simulink model "STATCOM_ssc_Ccode"  (R2024b)
settings: Solver=FixedStepDiscrete  StartTime=0.0  StopTime=2  FixedStep=Ts  RelTol=1e-3  EnableMultiTasking=on
PostLoadFcn:
  | Ts=25e-6; Rsnu=500; Csnu=0.1e-6;
InitFcn:
  | Ts=25e-6; Rsnu=500; Csnu=0.1e-6;
undefined symbols (not defined in the file): DiscIntNeverNeededParam
libraries: ee_lib x19, simetran x14, fl_lib x12, nesl_utility x12, spsSecondOrderFilterLib x3, spsabctodq0Lib x2, simulink x1, spsMeanVariableFrequencyLib x1
(part 2 of 3)

== system STATCOM_ssc_Ccode/STATCOM Controller/Firing Pulses Generator ==
  Alpha : Inport  PortDimensions=1
  Sigma : Inport  Port=2  PortDimensions=1
  wt : Inport  Port=3  PortDimensions=1
  D_Alpha : Inport  Port=4  PortDimensions=1
  " Deg->Rad" : Gain  Gain=pi/180  SaturateOnIntegerOverflow=on  OutDataTypeStr=Inherit: Same as input  ParamDataTypeStr=Inherit: Same as input
  Bridge 1D : Subsystem
  "Bridge 1Y " : Subsystem
  Bridge 2D : Subsystem
  Bridge 2Y : Subsystem
  Constant : Constant  Value=[0 -30 -15 -45]*pi/180 + 7.5*pi/180
  Deg->Rad : Gain  Gain=pi/180  SaturateOnIntegerOverflow=on  OutDataTypeStr=Inherit: Same as input  ParamDataTypeStr=Inherit: Same as input
  "Deg->Rad " : Gain  Gain=pi/180  SaturateOnIntegerOverflow=on  OutDataTypeStr=Inherit: Same as input  ParamDataTypeStr=Inherit: Same as input
  Demux : Demux
      settings: DisplayOption=none
  Mux : Mux  Inputs=[12 12 12 12]
  Sum : Sum  InputSameDT=on  SaturateOnIntegerOverflow=on  OutDataTypeStr=Inherit: Same as first input
  Pulses : Outport  VectorParamsAs1DForOutWhenUnconnected=off
  wires:
  wt/1 -> Sum/1
  Bridge 2D/1(Pulses) -> Mux/4
  Bridge 2Y/1(Pulses) -> Mux/3
  Bridge 1D/1(Pulses) -> Mux/2
  D_Alpha/1 -> " Deg->Rad"/1
  " Deg->Rad"/1 -> "Bridge 1Y "/4(D_Alpha), Bridge 1D/4(D_Alpha), Bridge 2Y/4(D_Alpha), Bridge 2D/4(D_Alpha)
  "Deg->Rad "/1 -> Bridge 2D/3(Sigma), Bridge 2Y/3(Sigma), Bridge 1D/3(Sigma), "Bridge 1Y "/3(Sigma)
  Deg->Rad/1 -> Bridge 2D/2(Alpha), Bridge 2Y/2(Alpha), Bridge 1D/2(Alpha), "Bridge 1Y "/2(Alpha)
  Demux/4 -> Bridge 2D/1(wt)
  Demux/3 -> Bridge 2Y/1(wt)
  Demux/2 -> Bridge 1D/1(wt)
  Sigma/1 -> "Deg->Rad "/1
  Demux/1 -> "Bridge 1Y "/1(wt)
  Mux/1 -> Pulses/1
  "Bridge 1Y "/1(Pulses) -> Mux/1
  Sum/1 -> Demux/1
  Constant/1 -> Sum/2
  Alpha/1 -> Deg->Rad/1

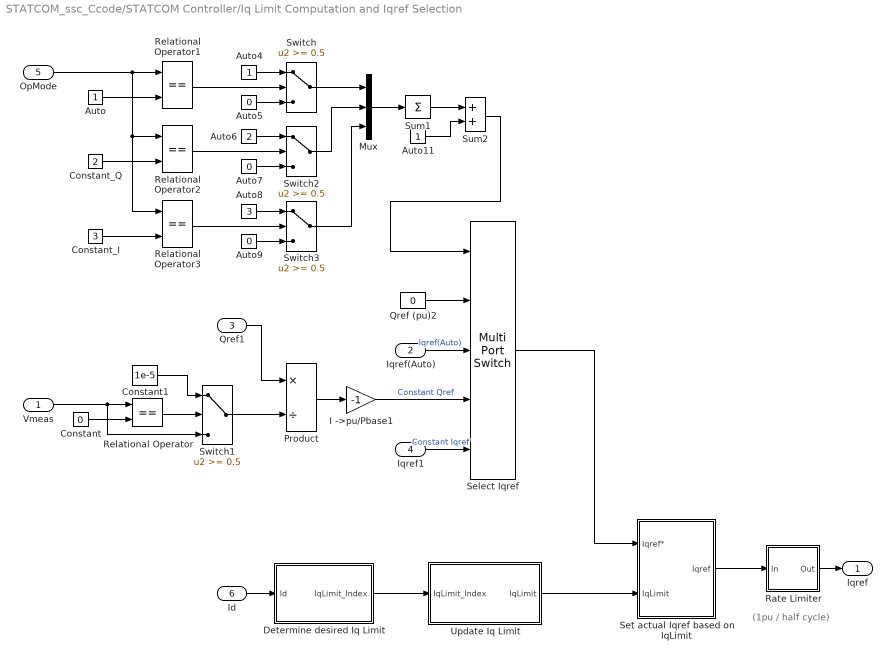
== system STATCOM_ssc_Ccode/STATCOM Controller/Iq Limit Computation and Iqref Selection ==
  note: (1pu / half cycle)
  Vmeas : Inport
  Iqref(Auto) : Inport  Port=2
  Qref1 : Inport  Port=3
  Iqref1 : Inport  Port=4
  OpMode : Inport  Port=5
  Id : Inport  Port=6
  Auto : Constant
  Auto11 : Constant
  Auto4 : Constant
  Auto5 : Constant  Value=0
  Auto6 : Constant  Value=2
  Auto7 : Constant  Value=0
  Auto8 : Constant  Value=3
  Auto9 : Constant  Value=0
  Constant : Constant  Value=0
  Constant1 : Constant  Value=1e-5
  Constant_I : Constant  Value=3
  Constant_Q : Constant  Value=2
  Determine desired Iq Limit : Subsystem
  I ->pu/Pbase1 : Gain  Gain=-1  SaturateOnIntegerOverflow=on  OutDataTypeStr=Inherit: Same as input  ParamDataTypeStr=Inherit: Same as input
  Mux : Mux  Inputs=3
  Product : Product  Inputs=*/  InputSameDT=on  SaturateOnIntegerOverflow=on  OutDataTypeStr=Inherit: Same as first input
  Qref (pu)2 : Constant  Value=0
  "Rate Limiter " : Subsystem  DialogController=POWERSYS.PowerSysDialog  mask(Discrete Rate Limiter){R=120, F=-120, Vinit=-0.33, Ts=Ts}
      mask prompts: R "Rising slew rate:"; F "Falling slew rate:"; Vinit "Initial input:"; Ts "Sample time:"
      mask help: DISCRETE BLOCK : Limit rising and falling rates of signal
      mask init:
      | UpperLimit=R*Ts;
      | LowerLimit=F*Ts;
      | power_initmask();
      mask Help: This block is part of a subset of blocks in the Extras library that does not have documentation associated with it, other than the block mask description.
      mask Display: disp('Discrete\nRate\nLimiter')
  Relational Operator{,1..3} (4 alike) : RelationalOperator  Operator===
  Select Iqref : MultiPortSwitch  Inputs=4
  Set actual Iqref based on IqLimit : Subsystem
  Sum1 : Sum  Inputs=1  InputSameDT=on  SaturateOnIntegerOverflow=on  OutDataTypeStr=Inherit: Same as first input
  Sum2 : Sum  InputSameDT=on  SaturateOnIntegerOverflow=on  OutDataTypeStr=Inherit: Same as first input
  Switch{,1..3} (4 alike) : Switch  Threshold=0.5
  Update Iq Limit : Subsystem
  Iqref : Outport  VectorParamsAs1DForOutWhenUnconnected=off
  wires:
  Id/1 -> Determine desired Iq Limit/1(Id)
  "Rate Limiter "/1(Out) -> Iqref/1
  Update Iq Limit/1(IqLimit) -> Set actual Iqref based on IqLimit/2(IqLimit)
  Determine desired Iq Limit/1(IqLimit_Index) -> Update Iq Limit/1(IqLimit_Index)
  Select Iqref/1 -> Set actual Iqref based on IqLimit/1(Iqref*)
  Qref (pu)2/1 -> Select Iqref/2
  I ->pu/Pbase1/1 -> Select Iqref/4  "Constant Qref"
  Iqref(Auto)/1 -> Select Iqref/3  "Iqref(Auto)"
  Iqref1/1 -> Select Iqref/5  "Constant Iqref"
  Product/1 -> I ->pu/Pbase1/1
  Constant/1 -> Relational Operator/2
  Switch1/1 -> Product/2
  Constant1/1 -> Switch1/1
  Relational Operator/1 -> Switch1/2
  Qref1/1 -> Product/1
  Vmeas/1 -> Switch1/3, Relational Operator/1
  Sum2/1 -> Select Iqref/1
  Auto/1 -> Relational Operator1/2
  Constant_Q/1 -> Relational Operator2/2
  Constant_I/1 -> Relational Operator3/2
  OpMode/1 -> Relational Operator1/1, Relational Operator2/1, Relational Operator3/1
  Relational Operator1/1 -> Switch/2
  Auto4/1 -> Switch/1
  Auto5/1 -> Switch/3
  Relational Operator2/1 -> Switch2/2
  Auto6/1 -> Switch2/1
  Auto7/1 -> Switch2/3
  Relational Operator3/1 -> Switch3/2
  Auto8/1 -> Switch3/1
  Auto9/1 -> Switch3/3
  Switch/1 -> Mux/1
  Mux/1 -> Sum1/1
  Switch3/1 -> Mux/3
  Sum1/1 -> Sum2/1
  Auto11/1 -> Sum2/2
  Switch2/1 -> Mux/2
  Set actual Iqref based on IqLimit/1(Iqref) -> "Rate Limiter "/1(In)

== system STATCOM_ssc_Ccode/STATCOM Controller/Measurement System ==
  Vabc : Inport  PortDimensions=3
  Iabc : Inport  Port=2  PortDimensions=3
  Freq : Inport  Port=3  PortDimensions=1
  wt : Inport  Port=4  PortDimensions=1
  Mean value : Subsystem  mask(Discrete Variable-Frequency Mean Value){Finit=60, Vinit=0, Ts=Ts}
      mask prompts: Finit "Initial Frequency (Hz):"; Vinit "Initial input (DC component):"; Ts "Sample time:"
      mask help:
      | This discrete block computes the mean value of the input signal (port In) over a running window of one cycle of a specified frequency (port Freq).
      |
      | For the first cycle of simulation (specified by the parameter "Initial frequency"), the output is held to the value of the  "Initial input" parameter.
  Mux : Mux  Inputs=2
  PQ Computaion : Subsystem
  Reactive current measurement (Iq) : Subsystem  mask(abc to dq0 Transformation){}
      mask help:
      | This block performs the  abc to dq0 transformation on a set of three-phase signals.
      |
      | It computes the three components ( Vd=direct axis , Vq=quadrature axis and V0=zero sequence) in a two axis rotating reference frame according to the following transformation:
      |
      | Vd = 2/3*[Va*sin(wt)  + Vb*sin(wt-2pi/3)  +  Vc*sin(wt+2pi/3)]
      | Vq = 2/3*[Va*cos(wt) + Vb*cos(wt-2pi/3) + Vc*cos(wt+2pi/3)]
      | V0 = 1/3*[Va +  Vb  +  Vc ]
      | where w=  rotation speed (rad/s) of the rotating frame.
      |
      | Input 1 contains  the vectorized  signals of the three  [Va Vb  Vc] sinusoidal phase quantities.
      | Input 2 must contain a  [sin(wt)  cos(wt)] two dimension signal , where w is the rotation speed (rad/s)  of the reference frame.
      | Output is a vectozized signal containing the [Vd Vq Vo] components.
      |
      | Press Help for more information.
      mask Help:
      | This transformation is commonly used in three-phase electric machine models where it is known as Park transformation. It allows to eliminate time varying inductances by referring the stator and rotor quantities to a fixed or rotating reference frame .
      | In case of a synchrounous machine, the stator quantities are referred to the rotor. Id and Iq represent the two DC currents flowing  in the two equivalent rotor windings ( d winding on the same axis as the field winding, and q winding in quadrature) producing the same flux as the stator Ia, Ib and Ic currents.
      | 
      | You can also use this block in a control system to measure the positive-sequence component V1 of a set of three-phase voltages or currents.
      | Vd and Vq represent the rectangular coordinates of  V1.
      | Use the Math Function block (hypot) and the Trigonometric function block (atan2) to obtain the modulus and angle of V1.
      | Mag(V1) = sqrt(Vd^2 + Vq^2);
      | Phase(V1)=atan2(Vq/Vd).
      | This measurement system does not introduce any delay, but, in contrast with the Fourier analysis (See Sequence Analyzer block), it is sensitive to harmonics and unbalances.
      | 
      | See also the dq0_to_abc block performing the reverse transformation.
  Second-Order Filter : spsSecondOrderFilterLib/Second-Order Filter  FilterType=Lowpass  Fo=1200  Zeta=0.707  Ts=Ts  Initialize=off  Vac_Init="[0,  0,  60]"  Vdc_Init=0  PlotResponse=off  FreqRange=[0, 500, 1]
  Second-Order Filter1 : spsSecondOrderFilterLib/Second-Order Filter  FilterType=Lowpass  Fo=1200  Zeta=0.707  Ts=Ts  Initialize=off  Vac_Init="[0,  0,  60]"  Vdc_Init=0  PlotResponse=off  FreqRange=[0, 500, 1]
  Selector : Selector  InputPortWidth=2  IndexOptions=Index vector (dialog)  Indices=2  OutputSizes=1
  Selector1 : Selector  InputPortWidth=2  IndexOptions=Index vector (dialog)  Indices=1  OutputSizes=1
  Trigonometric Function : Trigonometry
  Trigonometric Function1 : Trigonometry  Operator=cos
  Voltage measurement (Positive sequence) : Subsystem  mask(Discrete 3-phase PLL-Driven Positive-Sequence Fundamental Value){Finit=60, Par_Init=[1 0], Ts=Ts}
      mask prompts: Finit "Initial fundamental frequency (Hz):"; Par_Init "Initial input (positive component): [ Mag  Phase-relative-to-PLL(degrees) ]"; Ts "Sample time:"
      mask help:
      | For a supplied fundamental frequency (port Freq), this discrete block computes  the positive-sequence component (Magnitude and Phase)  of a set of three balanced or unbalanced signals (port abc) which may contain harmonics.
      |  Input port "Sin_Cos" (a two-dimension signal) provides the reference frame required for the computation..
      |  First and second outputs return respectively the magnitude and phase (in degrees relative to the PLL phase)) of the fundamental.
      | For the first cycle of simulation, the outputs are held constant to the values specified by the parameter "Initial input".
      mask init:
      | Real_Init=Par_Init(1)*cos(pi/180*Par_Init(2));
      | Imag_Init=Par_Init(1)*sin(pi/180*Par_Init(2));
  Vmeas : Outport  VectorParamsAs1DForOutWhenUnconnected=off
  PQ : Outport  Port=2  VectorParamsAs1DForOutWhenUnconnected=off
  Iq : Outport  Port=3  VectorParamsAs1DForOutWhenUnconnected=off
  Iq_avg : Outport  Port=4  VectorParamsAs1DForOutWhenUnconnected=off
  Id : Outport  Port=5  VectorParamsAs1DForOutWhenUnconnected=off
  wires:
  Second-Order Filter1/1 -> Iq/1
  Voltage measurement (Positive sequence)/2(VdVq) -> PQ Computaion/1(Vd_Vq)
  Voltage measurement (Positive sequence)/1(Mag) -> Vmeas/1  "Vmes"
  Vabc/1 -> Voltage measurement (Positive sequence)/1(abc)
  Trigonometric Function/1 -> Mux/1
  Trigonometric Function1/1 -> Mux/2
  wt/1 -> Trigonometric Function/1, Trigonometric Function1/1, Voltage measurement (Positive sequence)/3(wt)
  Iabc/1 -> Reactive current measurement (Iq)/2(abc)
  Mux/1 -> Reactive current measurement (Iq)/1(sin_cos)
  PQ Computaion/1(PQ(pu)) -> PQ/1
  Reactive current measurement (Iq)/1(IdIq) -> PQ Computaion/2(Id_Iq), Selector/1, Selector1/1
  Freq/1 -> Voltage measurement (Positive sequence)/2(Freq), PQ Computaion/3(Freq), Mean value/1(Freq)
  Selector/1 -> Mean value/2(In), Second-Order Filter1/1
  Mean value/1(Mean) -> Iq_avg/1
  Selector1/1 -> Second-Order Filter/1
  Second-Order Filter/1 -> Id/1

== system STATCOM_ssc_Ccode/STATCOM Controller/PLL ==
  Vabc (pu) : Inport  PortDimensions=3
  Constant4 : Constant  Value=2*pi
  Correction for delay : Gain  Gain=Nstep*Ts*2*pi  SaturateOnIntegerOverflow=on  OutDataTypeStr=Inherit: Same as input  ParamDataTypeStr=Inherit: Same as input
  Discrete PI Controller : Subsystem  DialogController=POWERSYS.PowerSysDialog  mask(Discrete PI Controller){Kp=Kp, Ki=Ki, Par_Limits=2*pi*Finit*[1.25 0.75], Init=2*pi*Finit, Ts=Ts}
      mask prompts: Kp "Proportional gain (Kp):"; Ki "Integral gain (Ki):"; Par_Limits "Output limits: [ Upper   Lower ]"; Init "Output initial value:"; Ts "Sample time:"
      mask help: This block implements a discrete PI controller.
      mask init:
      | UpperLimit=Par_Limits(1);
      | LowerLimit=Par_Limits(2);
      | power_initmask();
      mask Help: This block is part of a subset of blocks in the Extras library that does not have documentation associated with it, other than the block mask description.
      mask Display: disp('PI');
  Discrete Rate Limiter : Subsystem  DialogController=POWERSYS.PowerSysDialog  mask(Discrete Rate Limiter){R=10, F=-10, Vinit=Finit, Ts=Ts}
      mask prompts: R "Rising slew rate:"; F "Falling slew rate:"; Vinit "Initial input:"; Ts "Sample time:"
      mask help: DISCRETE BLOCK : Limit rising and falling rates of signal
      mask init:
      | UpperLimit=R*Ts;
      | LowerLimit=F*Ts;
      | power_initmask();
      mask Help: This block is part of a subset of blocks in the Extras library that does not have documentation associated with it, other than the block mask description.
      mask Display: disp('Discrete\nRate\nLimiter')
  Discrete-Time Integrator : DiscreteIntegrator  InitialCondition=Phase_Init*pi/180  SampleTime=Ts  ICPrevOutput=DiscIntNeverNeededParam  ICPrevScaledInput=DiscIntNeverNeededParam
  Gain10 : Gain  Gain=1/2/pi  SaturateOnIntegerOverflow=on  OutDataTypeStr=Inherit: Same as input  ParamDataTypeStr=Inherit: Same as input
  Math Function : Math  Operator=mod  SignedPower=on
  Mean (Variable Frequency) : spsMeanVariableFrequencyLib/Mean (Variable Frequency)  Finit=Finit  Fmin=45  Vinit=0  Ts=Ts
  Second-Order Filter : spsSecondOrderFilterLib/Second-Order Filter  FilterType=Lowpass  Fo=25  Zeta=0.707  Ts=Ts  Initialize=on  Vac_Init=[0 -25 60]  Vdc_Init=Finit  PlotResponse=off  FreqRange=[0, 500, 1]
  Selector : Selector  InputPortWidth=3  IndexOptions=Index vector (dialog)  Indices=2  OutputSizes=1
  Sum : Sum  InputSameDT=on  SaturateOnIntegerOverflow=on  OutDataTypeStr=Inherit: Same as first input
  Unit Delay : UnitDelay  InitialCondition=Finit  SampleTime=Ts  HasFrameUpgradeWarning=on
  abc to dq0 : spsabctodq0Lib/abc to dq0  Alignment=90 degrees behind phase A axis
  Freq : Outport  VectorParamsAs1DForOutWhenUnconnected=off
  wt : Outport  Port=2  VectorParamsAs1DForOutWhenUnconnected=off
  wires:
  Correction for delay/1 -> Sum/1
  Mean (Variable Frequency)/1 -> Discrete PI Controller/1(Error)
  Vabc (pu)/1 -> abc to dq0/1
  abc to dq0/1 -> Selector/1
  Constant4/1 -> Math Function/2
  Discrete-Time Integrator/1 -> Math Function/1
  Math Function/1 -> Sum/2, abc to dq0/2
  Discrete PI Controller/1(Out) -> Discrete-Time Integrator/1, Gain10/1  "W"
  Gain10/1 -> Discrete Rate Limiter/1(In)
  Discrete Rate Limiter/1(Out) -> Second-Order Filter/1
  Unit Delay/1 -> Freq/1, Mean (Variable Frequency)/1, Correction for delay/1
  Second-Order Filter/1 -> Unit Delay/1
  Selector/1 -> Mean (Variable Frequency)/2  "Vq"
  Sum/1 -> wt/1

== system STATCOM_ssc_Ccode/STATCOM Controller/Voltage Regulator ==
  Vref : Inport
  Vmeas : Inport  Port=2
  Discrete-Time Integrator : DiscreteIntegrator  InitialCondition=Init  SampleTime=Ts  LimitOutput=on  UpperSaturationLimit=UpperLimit  LowerSaturationLimit=LowerLimit  ICPrevOutput=DiscIntNeverNeededParam  ICPrevScaledInput=DiscIntNeverNeededParam
  Kp4 : Gain  Gain=Kp  SaturateOnIntegerOverflow=on  OutDataTypeStr=Inherit: Same as input  ParamDataTypeStr=Inherit: Same as input
  Kp5 : Gain  Gain=Ki  SaturateOnIntegerOverflow=on  OutDataTypeStr=Inherit: Same as input  ParamDataTypeStr=Inherit: Same as input
  Kp6 : Gain  Gain=Droop  SaturateOnIntegerOverflow=on  OutDataTypeStr=Inherit: Same as input  ParamDataTypeStr=Inherit: Same as input
  Saturation2 : Saturate  UpperLimit=UpperLimit  LowerLimit=LowerLimit
  Sum1 : Sum  Inputs=|-+  InputSameDT=on  SaturateOnIntegerOverflow=on  OutDataTypeStr=Inherit: Same as first input
  Sum6 : Sum  InputSameDT=on  SaturateOnIntegerOverflow=on  OutDataTypeStr=Inherit: Same as first input
  Sum7 : Sum  Inputs=|+-  InputSameDT=on  SaturateOnIntegerOverflow=on  OutDataTypeStr=Inherit: Same as first input
  Unit Delay : UnitDelay  SampleTime=Ts  HasFrameUpgradeWarning=on
  Iqref : Outport  InitialOutput=0  VectorParamsAs1DForOutWhenUnconnected=off
  wires:
  Discrete-Time Integrator/1 -> Sum6/2
  Kp4/1 -> Sum6/1
  Sum6/1 -> Saturation2/1
  Kp5/1 -> Discrete-Time Integrator/1
  Sum7/1 -> Kp5/1, Kp4/1
  Saturation2/1 -> Iqref/1, Kp6/1  "Iq_Ref"
  Kp6/1 -> Unit Delay/1
  Unit Delay/1 -> Sum7/2
  Vmeas/1 -> Sum1/1
  Vref/1 -> Sum1/2
  Sum1/1 -> Sum7/1  "Err"

== system STATCOM_ssc_Ccode/STATCOM Controller/DC Balance Regulator/ Mean value ==
  note: Discrete Mean Value
  note: Pierre Giroux, Gilbert Sybille
      | Power System Simulation Laboratory
      | IREQ, Hydro-Quebc
  In : Inport
  Constant : Constant  Value=Vinit
  Constant1 : Constant  Value=Correction
  Integ4 : DiscreteIntegrator  IntegratorMethod=Integration: Trapezoidal  SampleTime=Ts  ICPrevOutput=DiscIntNeverNeededParam  ICPrevScaledInput=DiscIntNeverNeededParam
  K2 : Constant  Value=Freq
  Product : Product  InputSameDT=on  SaturateOnIntegerOverflow=on  OutDataTypeStr=Inherit: Same as first input
  Product1 : Product  Inputs=**  InputSameDT=on  SaturateOnIntegerOverflow=on  OutDataTypeStr=Inherit: Same as first input
  Step : Step  Time=1/Freq  SampleTime=Ts
  Sum5 : Sum  InputSameDT=on  SaturateOnIntegerOverflow=on  OutDataTypeStr=Inherit: Same as first input
  Sum7 : Sum  Inputs=-+  InputSameDT=on  SaturateOnIntegerOverflow=on  OutDataTypeStr=Inherit: Same as first input
  Switch : Switch  Threshold=0.5
  Transport Delay : TransportDelay  DelayTime=Delay
  Mean : Outport  VectorParamsAs1DForOutWhenUnconnected=off
  wires:
  Switch/1 -> Mean/1
  Constant/1 -> Switch/3
  Step/1 -> Switch/2
  Sum5/1 -> Switch/1
  Product1/1 -> Sum5/2  "Correction"
  Constant1/1 -> Product1/2
  In/1 -> Product1/1, Integ4/1  "In"
  K2/1 -> Product/2
  Integ4/1 -> Sum7/2, Transport Delay/1
  Sum7/1 -> Product/1
  Transport Delay/1 -> Sum7/1
  Product/1 -> Sum5/1  "Mean value"

== system STATCOM_ssc_Ccode/STATCOM Controller/DC Balance Regulator/PI Regulator ==
  note: Discrete PID Controller
  note: Pierre Giroux, Gilbert Sybille
      | Power System Simulation Laboratory
      | IREQ, Hydro-Quebc
  Error : Inport
  Reset : Inport  Port=2
  Discrete-Time Integrator : DiscreteIntegrator  ExternalReset=rising  InitialCondition=Init  SampleTime=Ts  LimitOutput=on  UpperSaturationLimit=UpperLimit  LowerSaturationLimit=LowerLimit  ICPrevOutput=DiscIntNeverNeededParam  ICPrevScaledInput=DiscIntNeverNeededParam
  Kp4 : Gain  Gain=Kp  SaturateOnIntegerOverflow=on  OutDataTypeStr=Inherit: Same as input  ParamDataTypeStr=Inherit: Same as input
  Kp5 : Gain  Gain=Ki  SaturateOnIntegerOverflow=on  OutDataTypeStr=Inherit: Same as input  ParamDataTypeStr=Inherit: Same as input
  Saturation2 : Saturate  UpperLimit=UpperLimit  LowerLimit=LowerLimit
  Sum6 : Sum  InputSameDT=on  SaturateOnIntegerOverflow=on  OutDataTypeStr=Inherit: Same as first input
  Out : Outport  InitialOutput=0  VectorParamsAs1DForOutWhenUnconnected=off
  wires:
  Reset/1 -> Discrete-Time Integrator/2
  Error/1 -> Kp4/1, Kp5/1
  Sum6/1 -> Saturation2/1
  Kp5/1 -> Discrete-Time Integrator/1
  Kp4/1 -> Sum6/1
  Discrete-Time Integrator/1 -> Sum6/2
  Saturation2/1 -> Out/1

== system STATCOM_ssc_Ccode/STATCOM Controller/Firing Pulses Generator/Bridge 1D ==
  wt : Inport  PortDimensions=1
  Alpha : Inport  Port=2  PortDimensions=1
  Sigma : Inport  Port=3  PortDimensions=1
  D_Alpha : Inport  Port=4  PortDimensions=1
  Constant : Constant  Value=-2*pi/3
  Constant1 : Constant  Value=2*pi/3
  Mux1 : Mux  Inputs=[4 4 4]
  Phase A : Subsystem
  Phase B : Subsystem
  Phase C : Subsystem
  Sum : Sum  InputSameDT=on  SaturateOnIntegerOverflow=on  OutDataTypeStr=Inherit: Same as first input
  Sum1 : Sum  InputSameDT=on  SaturateOnIntegerOverflow=on  OutDataTypeStr=Inherit: Same as first input
  Sum2 : Sum  InputSameDT=on  SaturateOnIntegerOverflow=on  OutDataTypeStr=Inherit: Same as first input
  Pulses : Outport  VectorParamsAs1DForOutWhenUnconnected=off
  wires:
  Phase C/1(Pulses) -> Mux1/3
  Phase B/1(Pulses) -> Mux1/2
  D_Alpha/1 -> Phase C/3(D_Alpha), Phase B/3(D_Alpha), Phase A/3(D_Alpha)
  Sum1/1 -> Phase C/1(wt)
  Sum/1 -> Phase B/1(wt)
  Constant/1 -> Sum/2
  Phase A/1(Pulses) -> Mux1/1
  Mux1/1 -> Pulses/1
  Sum2/1 -> Sum1/1, Sum/1, Phase A/1(wt)
  wt/1 -> Sum2/1
  Alpha/1 -> Sum2/2
  Sigma/1 -> Phase B/2(sigma), Phase C/2(sigma), Phase A/2(sigma)
  Constant1/1 -> Sum1/2

== system STATCOM_ssc_Ccode/STATCOM Controller/Firing Pulses Generator/Bridge 1Y  ==
  wt : Inport  PortDimensions=1
  Alpha : Inport  Port=2  PortDimensions=1
  Sigma : Inport  Port=3  PortDimensions=1
  D_Alpha : Inport  Port=4  PortDimensions=1
  Constant : Constant  Value=-2*pi/3
  Constant1 : Constant  Value=2*pi/3
  Mux1 : Mux  Inputs=[4 4 4]
  Phase A : Subsystem
  Phase B : Subsystem
  Phase C : Subsystem
  Sum : Sum  InputSameDT=on  SaturateOnIntegerOverflow=on  OutDataTypeStr=Inherit: Same as first input
  Sum1 : Sum  InputSameDT=on  SaturateOnIntegerOverflow=on  OutDataTypeStr=Inherit: Same as first input
  Sum2 : Sum  InputSameDT=on  SaturateOnIntegerOverflow=on  OutDataTypeStr=Inherit: Same as first input
  Pulses : Outport  VectorParamsAs1DForOutWhenUnconnected=off
  wires:
  Constant1/1 -> Sum1/2
  Sigma/1 -> Phase A/2(sigma), Phase C/2(sigma), Phase B/2(sigma)
  Alpha/1 -> Sum2/2
  wt/1 -> Sum2/1
  Sum2/1 -> Phase A/1(wt), Sum/1, Sum1/1
  Mux1/1 -> Pulses/1
  Phase A/1(Pulses) -> Mux1/1
  Constant/1 -> Sum/2
  Sum/1 -> Phase B/1(wt)
  Sum1/1 -> Phase C/1(wt)
  D_Alpha/1 -> Phase A/3(D_Alpha), Phase B/3(D_Alpha), Phase C/3(D_Alpha)
  Phase B/1(Pulses) -> Mux1/2
  Phase C/1(Pulses) -> Mux1/3

== system STATCOM_ssc_Ccode/STATCOM Controller/Firing Pulses Generator/Bridge 2D ==
  wt : Inport  PortDimensions=1
  Alpha : Inport  Port=2  PortDimensions=1
  Sigma : Inport  Port=3  PortDimensions=1
  D_Alpha : Inport  Port=4  PortDimensions=1
  Constant : Constant  Value=-2*pi/3
  Constant1 : Constant  Value=2*pi/3
  Mux1 : Mux  Inputs=[4 4 4]
  Phase A : Subsystem
  Phase B : Subsystem
  Phase C : Subsystem
  Sum : Sum  InputSameDT=on  SaturateOnIntegerOverflow=on  OutDataTypeStr=Inherit: Same as first input
  Sum1 : Sum  InputSameDT=on  SaturateOnIntegerOverflow=on  OutDataTypeStr=Inherit: Same as first input
  Sum2 : Sum  InputSameDT=on  SaturateOnIntegerOverflow=on  OutDataTypeStr=Inherit: Same as first input
  Pulses : Outport  VectorParamsAs1DForOutWhenUnconnected=off
  wires:
  Phase C/1(Pulses) -> Mux1/3
  Phase B/1(Pulses) -> Mux1/2
  D_Alpha/1 -> Phase C/3(D_Alpha), Phase B/3(D_Alpha), Phase A/3(D_Alpha)
  Sum1/1 -> Phase C/1(wt)
  Sum/1 -> Phase B/1(wt)
  Constant/1 -> Sum/2
  Phase A/1(Pulses) -> Mux1/1
  Mux1/1 -> Pulses/1
  Sum2/1 -> Sum1/1, Sum/1, Phase A/1(wt)
  wt/1 -> Sum2/1
  Alpha/1 -> Sum2/2
  Sigma/1 -> Phase B/2(sigma), Phase C/2(sigma), Phase A/2(sigma)
  Constant1/1 -> Sum1/2

== system STATCOM_ssc_Ccode/STATCOM Controller/Firing Pulses Generator/Bridge 2Y ==
  wt : Inport  PortDimensions=1
  Alpha : Inport  Port=2  PortDimensions=1
  Sigma : Inport  Port=3  PortDimensions=1
  D_Alpha : Inport  Port=4  PortDimensions=1
  Constant : Constant  Value=-2*pi/3
  Constant1 : Constant  Value=2*pi/3
  Mux1 : Mux  Inputs=[4 4 4]
  Phase A : Subsystem
  Phase B : Subsystem
  Phase C : Subsystem
  Sum : Sum  InputSameDT=on  SaturateOnIntegerOverflow=on  OutDataTypeStr=Inherit: Same as first input
  Sum1 : Sum  InputSameDT=on  SaturateOnIntegerOverflow=on  OutDataTypeStr=Inherit: Same as first input
  Sum2 : Sum  InputSameDT=on  SaturateOnIntegerOverflow=on  OutDataTypeStr=Inherit: Same as first input
  Pulses : Outport  VectorParamsAs1DForOutWhenUnconnected=off
  wires:
  Constant1/1 -> Sum1/2
  Sigma/1 -> Phase A/2(sigma), Phase C/2(sigma), Phase B/2(sigma)
  Alpha/1 -> Sum2/2
  wt/1 -> Sum2/1
  Sum2/1 -> Phase A/1(wt), Sum/1, Sum1/1
  Mux1/1 -> Pulses/1
  Phase A/1(Pulses) -> Mux1/1
  Constant/1 -> Sum/2
  Sum/1 -> Phase B/1(wt)
  Sum1/1 -> Phase C/1(wt)
  D_Alpha/1 -> Phase A/3(D_Alpha), Phase B/3(D_Alpha), Phase C/3(D_Alpha)
  Phase B/1(Pulses) -> Mux1/2
  Phase C/1(Pulses) -> Mux1/3

== system STATCOM_ssc_Ccode/STATCOM Controller/Iq Limit Computation and Iqref Selection/Determine desired Iq Limit ==
  note: Determine desired Iq Limit (by step of 0.1 pu, from 1 to 0.3 pu)
      | based on actual value of Id
      | 5% above rated current is allowed
      | i.e.   sqrt ( Id^2 + Iq^2 ) < 1.05 pu
  Id : Inport  PortDimensions=1
  Abs : Abs
  Constant : Constant
  Limit at 0.3 : Relay  OnSwitchValue=0.97  OffSwitchValue=0.92
  Limit at 0.4 : Relay  OnSwitchValue=0.92  OffSwitchValue=0.86
  Limit at 0.5 : Relay  OnSwitchValue=0.86  OffSwitchValue=0.78
  Limit at 0.6 : Relay  OnSwitchValue=0.78  OffSwitchValue=0.68
  Limit at 0.7 : Relay  OnSwitchValue=0.68  OffSwitchValue=0.54
  Limit at 0.8 : Relay  OnSwitchValue=0.54  OffSwitchValue=0.32
  Limit at 0.9 : Relay  OnSwitchValue=0.32  OffSwitchValue=0.25
  Sum : Sum  Inputs=++++++++  InputSameDT=on  SaturateOnIntegerOverflow=on  OutDataTypeStr=Inherit: Same as first input
  IqLimit_Index : Outport  VectorParamsAs1DForOutWhenUnconnected=off
  wires:
  Sum/1 -> IqLimit_Index/1
  Limit at 0.9/1 -> Sum/2
  Limit at 0.8/1 -> Sum/3
  Limit at 0.7/1 -> Sum/4
  Limit at 0.6/1 -> Sum/5
  Constant/1 -> Sum/1
  Id/1 -> Abs/1
  Abs/1 -> Limit at 0.9/1, Limit at 0.8/1, Limit at 0.7/1, Limit at 0.6/1, Limit at 0.5/1, Limit at 0.4/1, Limit at 0.3/1
  Limit at 0.5/1 -> Sum/6
  Limit at 0.4/1 -> Sum/7
  Limit at 0.3/1 -> Sum/8

== system STATCOM_ssc_Ccode/STATCOM Controller/Iq Limit Computation and Iqref Selection/Rate Limiter  ==
  note: Delta(u)
  note: Beat Ronner
      | ABB Industrie AG
      | Turgi, Switzerland
  In : Inport
  Saturation : Saturate  UpperLimit=UpperLimit  LowerLimit=LowerLimit
  Sum : Sum  Inputs=|++  InputSameDT=on  SaturateOnIntegerOverflow=on  OutDataTypeStr=Inherit: Same as first input
  Sum1 : Sum  Inputs=|+-  InputSameDT=on  SaturateOnIntegerOverflow=on  OutDataTypeStr=Inherit: Same as first input
  Unit Delay : UnitDelay  InitialCondition=Vinit  SampleTime=Ts  HasFrameUpgradeWarning=on
  Out : Outport  VectorParamsAs1DForOutWhenUnconnected=off
  wires:
  In/1 -> Sum1/1  "u"
  Sum1/1 -> Saturation/1
  Saturation/1 -> Sum/1  "Delta(u)_limit"
  Sum/1 -> Out/1, Unit Delay/1  "y"
  Unit Delay/1 -> Sum1/2, Sum/2  "y-1"

== system STATCOM_ssc_Ccode/STATCOM Controller/Iq Limit Computation and Iqref Selection/Set actual Iqref based on IqLimit ==
  Iqref* : Inport  PortDimensions=1
  IqLimit : Inport  Port=2
  Gain2 : Gain  Gain=-1  SaturateOnIntegerOverflow=on  OutDataTypeStr=Inherit: Same as input  ParamDataTypeStr=Inherit: Same as input
  Logical Operator : Logic  Operator=OR
  Product : Product  InputSameDT=on  SaturateOnIntegerOverflow=on  OutDataTypeStr=Inherit: Same as first input
  Relational Operator1 : RelationalOperator  Operator=>
  Relational Operator2 : RelationalOperator  Operator=<
  Sign : Signum
  Switch1 : Switch  Threshold=0.5
  Iqref : Outport  VectorParamsAs1DForOutWhenUnconnected=off
  wires:
  Switch1/1 -> Iqref/1
  IqLimit/1 -> Product/1, Relational Operator1/2, Gain2/1
  Gain2/1 -> Relational Operator2/2
  Relational Operator1/1 -> Logical Operator/1
  Relational Operator2/1 -> Logical Operator/2
  Logical Operator/1 -> Switch1/2
  Iqref*/1 -> Relational Operator1/1, Relational Operator2/1, Switch1/3, Sign/1
  Sign/1 -> Product/2
  Product/1 -> Switch1/1

== system STATCOM_ssc_Ccode/STATCOM Controller/Iq Limit Computation and Iqref Selection/Update Iq Limit ==
  note: 2) Update of the new desired Iq limit is delayed by 3 cycles if the new desired limit is higher then the actual limit
  note: Rules for updating the Iq Limit in order to avoid control instability :
  note: 1) Instantaneous update of IqLimit if the new desired Iq limit is lower then the actual limit
  IqLimit_Index : Inport
  Constant1 : Constant  Value=0.8
  Constant10 : Constant  Value=-1e6
  Constant11 : Constant  Value=3
  Constant2 : Constant  Value=0.7
  Constant3 : Constant  Value=0.6
  Constant4 : Constant  Value=0.5
  Constant5 : Constant  Value=0.4
  Constant6 : Constant
  Constant7 : Constant  Value=0.9
  Constant8 : Constant  Value=0.3
  Constant9 : Constant  Value=60
  Discrete-Time Integrator : DiscreteIntegrator  ExternalReset=rising  SampleTime=Ts  LimitOutput=on  UpperSaturationLimit=6.1  LowerSaturationLimit=0  ICPrevOutput=DiscIntNeverNeededParam  ICPrevScaledInput=DiscIntNeverNeededParam
  Logical Operator1 : Logic  Operator=OR
  Relational Operator3 : RelationalOperator  Operator=>
  Relational Operator4 : RelationalOperator  Operator=>
  Relational Operator5 : RelationalOperator  Operator=<
  Select actual Iq Limit : MultiPortSwitch  Inputs=8
  Switch : Switch  Threshold=0.5
  Switch2 : Switch  Threshold=0.5
  Unit Delay : UnitDelay  SampleTime=Ts  HasFrameUpgradeWarning=on
  Unit Delay5 : UnitDelay  InitialCondition=1  SampleTime=Ts  HasFrameUpgradeWarning=on
  IqLimit : Outport  VectorParamsAs1DForOutWhenUnconnected=off
  wires:
  IqLimit_Index/1 -> Relational Operator5/2, Relational Operator3/2, Switch2/1
  Relational Operator5/1 -> Logical Operator1/2
  Relational Operator4/1 -> Logical Operator1/1, Unit Delay/1
  Discrete-Time Integrator/1 -> Relational Operator4/1
  Constant11/1 -> Relational Operator4/2
  Switch/1 -> Discrete-Time Integrator/1
  Unit Delay/1 -> Discrete-Time Integrator/2
  Constant9/1 -> Switch/1
  Constant10/1 -> Switch/3
  Relational Operator3/1 -> Switch/2
  Unit Delay5/1 -> Relational Operator5/1, Relational Operator3/1, Switch2/3, Select actual Iq Limit/1
  Switch2/1 -> Unit Delay5/1
  Logical Operator1/1 -> Switch2/2
  Select actual Iq Limit/1 -> IqLimit/1
  Constant3/1 -> Select actual Iq Limit/6
  Constant2/1 -> Select actual Iq Limit/5
  Constant1/1 -> Select actual Iq Limit/4
  Constant7/1 -> Select actual Iq Limit/3
  Constant6/1 -> Select actual Iq Limit/2
  Constant8/1 -> Select actual Iq Limit/9
  Constant5/1 -> Select actual Iq Limit/8
  Constant4/1 -> Select actual Iq Limit/7

== system STATCOM_ssc_Ccode/STATCOM Controller/Measurement System/Mean value ==
  note: Pierre Giroux, Gilbert Sybille
      | Power System Simulation Laboratory
      | IREQ, Hydro-Quebc
  note: Variable frequency - Discrete Mean Value
  Freq : Inport
  In : Inport  Port=2
  Constant : Constant  Value=Vinit
  Gain : Gain  Gain=Ts  SaturateOnIntegerOverflow=on  OutDataTypeStr=Inherit: Same as input  ParamDataTypeStr=Inherit: Same as input
  Integ4 : DiscreteIntegrator  IntegratorMethod=Integration: Trapezoidal  SampleTime=Ts  ICPrevOutput=DiscIntNeverNeededParam  ICPrevScaledInput=DiscIntNeverNeededParam
  K2 : Constant  Value=Ts/2
  Number of sample/cycle : Fcn  Expr=1/(u[1]+1e-6)/Ts
  Product : Product  InputSameDT=on  SaturateOnIntegerOverflow=on  OutDataTypeStr=Inherit: Same as first input
  Product1 : Product  Inputs=*/*  InputSameDT=on  SaturateOnIntegerOverflow=on  OutDataTypeStr=Inherit: Same as first input
  Rounding Function : Rounding  Operator=round
  Step : Step  Time=1/Finit  SampleTime=Ts
  Sum3 : Sum  Inputs=-+  InputSameDT=on  SaturateOnIntegerOverflow=on  OutDataTypeStr=Inherit: Same as first input
  Sum4 : Sum  Inputs=-+  InputSameDT=on  SaturateOnIntegerOverflow=on  OutDataTypeStr=Inherit: Same as first input
  Sum5 : Sum  InputSameDT=on  SaturateOnIntegerOverflow=on  OutDataTypeStr=Inherit: Same as first input
  Sum7 : Sum  Inputs=-+  InputSameDT=on  SaturateOnIntegerOverflow=on  OutDataTypeStr=Inherit: Same as first input
  Switch : Switch  Threshold=0.5
  Variable Transport Delay2 : VariableTransportDelay  MaximumDelay=20e-3
  Mean : Outport  VectorParamsAs1DForOutWhenUnconnected=off
  wires:
  Product1/1 -> Sum5/2  "Correction"
  In/1 -> Product1/3, Integ4/1  "In"
  Product/1 -> Sum5/1  "Mean value"
  Variable Transport Delay2/1 -> Sum7/1
  Sum7/1 -> Product/1
  Integ4/1 -> Variable Transport Delay2/1, Sum7/2
  Freq/1 -> Product/2, Number of sample/cycle/1  "Freq"
  K2/1 -> Sum3/1
  Gain/1 -> Sum3/2
  Rounding Function/1 -> Gain/1, Product1/2, Sum4/1
  Sum4/1 -> Product1/1
  Number of sample/cycle/1 -> Rounding Function/1, Sum4/2
  Sum3/1 -> Variable Transport Delay2/2  "Delay"
  Sum5/1 -> Switch/1
  Step/1 -> Switch/2
  Constant/1 -> Switch/3
  Switch/1 -> Mean/1

== system STATCOM_ssc_Ccode/STATCOM Controller/Measurement System/PQ Computaion ==
  note: P = Vd*Id + Vq*Iq
  note: Q = Vq*Id-Vd*Iq
  note: PQ Measurement:
  Vd_Vq : Inport  PortDimensions=2
  Id_Iq : Inport  Port=2  PortDimensions=2
  Freq : Inport  Port=3  PortDimensions=1
  Demux1 : Demux  Outputs=2
      settings: DisplayOption=none
  Demux2 : Demux  Outputs=2
      settings: DisplayOption=none
  Mux2 : Mux  Inputs=2
  Product{2..5} (4 alike) : Product  InputSameDT=on  SaturateOnIntegerOverflow=on  OutDataTypeStr=Inherit: Same as first input
  Sum : Sum  InputSameDT=on  SaturateOnIntegerOverflow=on  OutDataTypeStr=Inherit: Same as first input
  Sum1 : Sum  Inputs=+-  InputSameDT=on  SaturateOnIntegerOverflow=on  OutDataTypeStr=Inherit: Same as first input
  Variable Frequency Mean value : Subsystem  mask(Discrete Variable-Frequency Mean Value){Finit=60, Vinit=0, Ts=Ts}
      mask prompts: Finit "Initial Frequency (Hz):"; Vinit "Initial input (DC component):"; Ts "Sample time:"
      mask help:
      | This discrete block computes the mean value of the input signal (port In) over a running window of one cycle of a specified frequency (port Freq).
      |
      | For the first cycle of simulation (specified by the parameter "Initial frequency"), the output is held to the value of the  "Initial input" parameter.
  PQ(pu) : Outport  VectorParamsAs1DForOutWhenUnconnected=off
  wires:
  Product2/1 -> Sum/1
  Product3/1 -> Sum/2
  Product4/1 -> Sum1/1
  Product5/1 -> Sum1/2
  Sum/1 -> Mux2/1
  Sum1/1 -> Mux2/2
  Demux1/2 -> Product3/1, Product4/1
  Demux2/1 -> Product2/2, Product4/2
  Demux1/1 -> Product2/1, Product5/1
  Demux2/2 -> Product3/2, Product5/2
  Mux2/1 -> Variable Frequency Mean value/2(In)
  Variable Frequency Mean value/1(Mean) -> PQ(pu)/1
  Freq/1 -> Variable Frequency Mean value/1(Freq)
  Id_Iq/1 -> Demux2/1
  Vd_Vq/1 -> Demux1/1

== system STATCOM_ssc_Ccode/STATCOM Controller/Measurement System/Reactive current measurement (Iq) ==
  note: V0= 1/3 (Va + Vb + Vc )
  note: Vd= 2/3 (Va*sinwt + Vb*sin(wt-2pi/3) + Vc*sin(wt+2pi/3)
  note: sin
  note: cos
  note: cos
  note: Vq= 2/3 (Va*coswt + Vb*cos(wt-2pi/3) + Vc*cos(wt+2pi/3)
  sin_cos : Inport
  abc : Inport  Port=2
  Demux : Demux  Outputs=2
      settings: DisplayOption=none
  Fcn1 : Fcn  Expr=2/3*((u[1]*u[5])+(u[2]*u[7])+(u[3]*u[9]))
  Fcn2 : Fcn  Expr=2/3*((u[1]*u[4])+(u[2]*u[6])+(u[3]*u[8]))
  K1 : Constant  Value=0.5
  K2 : Constant  Value=sqrt(3)/2
  Mux : Mux  Inputs=2
  Mux1 : Mux  Inputs=2
  Mux2 : Mux  Inputs=6
  Product{,1..3} (4 alike) : Product  InputSameDT=on  SaturateOnIntegerOverflow=on  OutDataTypeStr=Inherit: Same as first input
  Sum : Sum  Inputs=--  InputSameDT=on  SaturateOnIntegerOverflow=on  OutDataTypeStr=Inherit: Same as first input
  Sum1 : Sum  Inputs=-+  InputSameDT=on  SaturateOnIntegerOverflow=on  OutDataTypeStr=Inherit: Same as first input
  Sum2 : Sum  Inputs=--  InputSameDT=on  SaturateOnIntegerOverflow=on  OutDataTypeStr=Inherit: Same as first input
  Sum3 : Sum  Inputs=--  InputSameDT=on  SaturateOnIntegerOverflow=on  OutDataTypeStr=Inherit: Same as first input
  IdIq : Outport  InitialOutput=0  VectorParamsAs1DForOutWhenUnconnected=off
  wires:
  Sum1/1 -> Sum3/1, Mux2/4  "cos(wt-2pi/3)"
  Sum/1 -> Sum2/1, Mux2/3  "sin(wt-2pi/3)"
  K2/1 -> Product2/2, Product1/2
  K1/1 -> Product3/2, Product/2
  Sum2/1 -> Mux2/5  "sin(wt+2pi/3)"
  Sum3/1 -> Mux2/6  "cos(wt+2pi/3)"
  Product2/1 -> Sum1/2
  Product3/1 -> Sum1/1
  Product1/1 -> Sum/2
  Product/1 -> Sum/1
  Demux/1 -> Mux2/1, Sum2/2, Product2/1, Product/1  "sin(wt)"
  Demux/2 -> Mux2/2, Product1/1, Product3/1, Sum3/2  "cos(wt)"
  sin_cos/1 -> Demux/1
  Mux2/1 -> Mux/2
  abc/1 -> Mux/1  "Vabc"
  Mux/1 -> Fcn1/1, Fcn2/1
  Fcn2/1 -> Mux1/1  "Id"
  Fcn1/1 -> Mux1/2  "Iq"
  Mux1/1 -> IdIq/1

== system STATCOM_ssc_Ccode/STATCOM Controller/Measurement System/Voltage measurement (Positive sequence) ==
  note: Discrete 3-phase PLL-Driven Positive-Sequence Fundamental Value
  note: Pierre Giroux, Gilbert Sybille
      | Power System Simulation Laboratory
      | IREQ, Hydro-Quebc
  abc : Inport  PortDimensions=3
  Freq : Inport  Port=2
  wt : Inport  Port=3  PortDimensions=1
  Demux : Demux  Outputs=3
      settings: DisplayOption=none
  Discrete Variable Frequency Mean value1 : Subsystem  mask(Discrete Variable-Frequency Mean Value){Finit=Finit, Vinit=Real_Init, Ts=Ts}
      mask prompts: Finit "Initial Frequency (Hz):"; Vinit "Initial input (DC component):"; Ts "Sample time:"
      mask help:
      | This discrete block computes the mean value of the input signal (port In) over a running window of one cycle of a specified frequency (port Freq).
      |
      | For the first cycle of simulation (specified by the parameter "Initial frequency"), the output is held to the value of the  "Initial input" parameter.
  Discrete Variable Frequency Mean value2 : Subsystem  mask(Discrete Variable-Frequency Mean Value){Finit=Finit, Vinit=Imag_Init, Ts=Ts}
      mask prompts: Finit "Initial Frequency (Hz):"; Vinit "Initial input (DC component):"; Ts "Sample time:"
      mask help:
      | This discrete block computes the mean value of the input signal (port In) over a running window of one cycle of a specified frequency (port Freq).
      |
      | For the first cycle of simulation (specified by the parameter "Initial frequency"), the output is held to the value of the  "Initial input" parameter.
  Fcn3 : Fcn  Expr=sqrt(u[1]*u[1]+u[2]*u[2])
  Mux1 : Mux  Inputs=2
  Selector : Selector  InputPortWidth=3  IndexOptions=Index vector (dialog)  Indices=[1 2]  OutputSizes=1
  Terminator : Terminator
  abc to dq0 : spsabctodq0Lib/abc to dq0  Alignment=90 degrees behind phase A axis
  Mag : Outport  VectorParamsAs1DForOutWhenUnconnected=off
  VdVq : Outport  Port=2  VectorParamsAs1DForOutWhenUnconnected=off
  wires:
  Demux/3 -> Terminator/1
  abc/1 -> abc to dq0/1
  Demux/1 -> Discrete Variable Frequency Mean value1/2(In)
  Demux/2 -> Discrete Variable Frequency Mean value2/2(In)
  Discrete Variable Frequency Mean value2/1(Mean) -> Mux1/2  "Real"
  Fcn3/1 -> Mag/1
  Discrete Variable Frequency Mean value1/1(Mean) -> Mux1/1  "Real"
  Freq/1 -> Discrete Variable Frequency Mean value1/1(Freq), Discrete Variable Frequency Mean value2/1(Freq)
  wt/1 -> abc to dq0/2
  abc to dq0/1 -> Demux/1, Selector/1
  Selector/1 -> VdVq/1
  Mux1/1 -> Fcn3/1

== system STATCOM_ssc_Ccode/STATCOM Controller/PLL/Discrete PI Controller ==
  note: Pierre Giroux, Gilbert Sybille
      | Power System Simulation Laboratory
      | IREQ, Hydro-Quebc
  note: Discrete PID Controller
  Error : Inport  SampleTime=Ts
  Discrete-Time Integrator : DiscreteIntegrator  InitialCondition=Init  SampleTime=Ts  LimitOutput=on  UpperSaturationLimit=UpperLimit  LowerSaturationLimit=LowerLimit  ICPrevOutput=DiscIntNeverNeededParam  ICPrevScaledInput=DiscIntNeverNeededParam
  Kp4 : Gain  Gain=Kp  SaturateOnIntegerOverflow=on  SampleTime=Ts  OutDataTypeStr=Inherit: Same as input  ParamDataTypeStr=Inherit: Same as input
  Kp5 : Gain  Gain=Ki  SaturateOnIntegerOverflow=on  SampleTime=Ts  OutDataTypeStr=Inherit: Same as input  ParamDataTypeStr=Inherit: Same as input
  Saturation2 : Saturate  UpperLimit=UpperLimit  LowerLimit=LowerLimit  SampleTime=Ts
  Sum6 : Sum  InputSameDT=on  SaturateOnIntegerOverflow=on  SampleTime=Ts  OutDataTypeStr=Inherit: Same as first input
  Zero-Order Hold : ZeroOrderHold  SampleTime=Ts
  Out : Outport  SampleTime=Ts  InitialOutput=0  VectorParamsAs1DForOutWhenUnconnected=off
  wires:
  Error/1 -> Kp4/1, Kp5/1
  Sum6/1 -> Saturation2/1
  Kp5/1 -> Discrete-Time Integrator/1
  Kp4/1 -> Zero-Order Hold/1
  Discrete-Time Integrator/1 -> Sum6/2
  Saturation2/1 -> Out/1
  Zero-Order Hold/1 -> Sum6/1

== system STATCOM_ssc_Ccode/STATCOM Controller/PLL/Discrete Rate Limiter ==
  note: Delta(u)
  note: Beat Ronner
      | ABB Industrie AG
      | Turgi, Switzerland
  In : Inport
  Saturation : Saturate  UpperLimit=UpperLimit  LowerLimit=LowerLimit
  Sum : Sum  Inputs=|++  InputSameDT=on  SaturateOnIntegerOverflow=on  OutDataTypeStr=Inherit: Same as first input
  Sum1 : Sum  Inputs=|+-  InputSameDT=on  SaturateOnIntegerOverflow=on  OutDataTypeStr=Inherit: Same as first input
  Unit Delay : UnitDelay  InitialCondition=Vinit  SampleTime=Ts  HasFrameUpgradeWarning=on
  Out : Outport  VectorParamsAs1DForOutWhenUnconnected=off
  wires:
  In/1 -> Sum1/1  "u"
  Sum1/1 -> Saturation/1
  Saturation/1 -> Sum/1  "Delta(u)_limit"
  Sum/1 -> Out/1, Unit Delay/1  "y"
  Unit Delay/1 -> Sum1/2, Sum/2  "y-1"

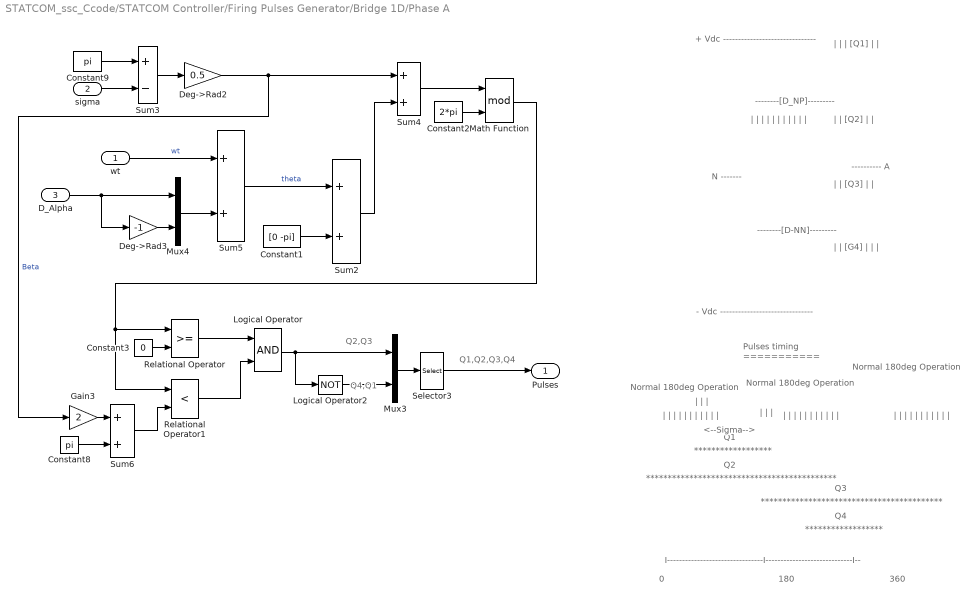
== system STATCOM_ssc_Ccode/STATCOM Controller/Firing Pulses Generator/Bridge 1D/Phase A ==
  note: |
      | |
      | |
      | [Q1]
      | |
      | |
  note: |
      | |
      | [Q2]
      | |
      | |
  note: |
      | |
      | [Q3]
      | |
      | |
  note: |
      | |
      | [G4]
      | |
      | |
      | |
  note: --------[D_NP]---------
  note: --------[D-NN]---------
  note: ---------- A
  note: |
      | |
      | |
      | |
      | |
      | |
      | |
      | |
      | |
      | |
      | |
  note: N -------
  note: - Vdc -------------------------------
  note: + Vdc -------------------------------
  note: Q4,Q1
  note: Q2,Q3
  note: Q1,Q2,Q3,Q4
  note: |
      | |
      | |
      | |
      | |
      | |
      | |
      | |
      | |
      | |
      | |
  note: |
      | |
      | |
      | |
      | |
      | |
      | |
      | |
      | |
      | |
      | |
  note: |
      | |
      | |
      | |
      | |
      | |
      | |
      | |
      | |
      | |
      | |
  note: Pulses timing
      | ===========
  note: Normal 180deg
      | Operation
  note: Normal 180deg
      | Operation
  note: Normal 180deg
      | Operation
  note: I--------------------------------I-----------------------------I--
  note: 0
  note: 180
  note: 360
  note: ******************
  note: ******************
  note: ********************************************
  note: ******************************************
  note: Q1
  note: Q2
  note: Q3
  note: Q4
  note: |
      | |
      | |
  note: |
      | |
      | |
  note: <--Sigma-->
  wt : Inport  PortDimensions=1
  sigma : Inport  Port=2  PortDimensions=1
  D_Alpha : Inport  Port=3  PortDimensions=1
  Constant1 : Constant  Value=[0 -pi]
  Constant2 : Constant  Value=2*pi
  Constant3 : Constant  Value=0
  Constant8 : Constant  Value=pi
  Constant9 : Constant  Value=pi
  Deg->Rad2 : Gain  Gain=0.5  SaturateOnIntegerOverflow=on  OutDataTypeStr=Inherit: Same as input  ParamDataTypeStr=Inherit: Same as input
  Deg->Rad3 : Gain  Gain=-1  SaturateOnIntegerOverflow=on  OutDataTypeStr=Inherit: Same as input  ParamDataTypeStr=Inherit: Same as input
  Gain3 : Gain  Gain=2  SaturateOnIntegerOverflow=on  OutDataTypeStr=Inherit: Same as input  ParamDataTypeStr=Inherit: Same as input
  Logical Operator : Logic
  Logical Operator2 : Logic  Operator=NOT
  Math Function : Math  Operator=mod  SignedPower=on
  Mux3 : Mux  Inputs=[2 2]
  Mux4 : Mux  Inputs=2
  Relational Operator : RelationalOperator
  Relational Operator1 : RelationalOperator  Operator=<
  Selector3 : Selector  InputPortWidth=4  IndexOptions=Index vector (dialog)  Indices=[4 1 2 3]  OutputSizes=1
  Sum{2,4..6} (4 alike) : Sum  InputSameDT=on  SaturateOnIntegerOverflow=on  OutDataTypeStr=Inherit: Same as first input
  Sum3 : Sum  Inputs=+-  InputSameDT=on  SaturateOnIntegerOverflow=on  OutDataTypeStr=Inherit: Same as first input
  Pulses : Outport  VectorParamsAs1DForOutWhenUnconnected=off
  wires:
  Constant1/1 -> Sum2/2
  Constant3/1 -> Relational Operator/2
  Relational Operator/1 -> Logical Operator/1
  Relational Operator1/1 -> Logical Operator/2
  Constant9/1 -> Sum3/1
  sigma/1 -> Sum3/2
  Sum3/1 -> Deg->Rad2/1
  Deg->Rad2/1 -> Sum4/1, Gain3/1  "Beta"
  Constant8/1 -> Sum6/2
  Sum6/1 -> Relational Operator1/2
  Sum2/1 -> Sum4/2
  Sum4/1 -> Math Function/1
  Logical Operator/1 -> Logical Operator2/1, Mux3/1
  Logical Operator2/1 -> Mux3/2
  Mux3/1 -> Selector3/1
  Selector3/1 -> Pulses/1
  Gain3/1 -> Sum6/1
  Math Function/1 -> Relational Operator1/1, Relational Operator/1
  Mux4/1 -> Sum5/2
  Deg->Rad3/1 -> Mux4/2
  D_Alpha/1 -> Deg->Rad3/1, Mux4/1
  wt/1 -> Sum5/1  "wt"
  Sum5/1 -> Sum2/1  "theta"
  Constant2/1 -> Math Function/2

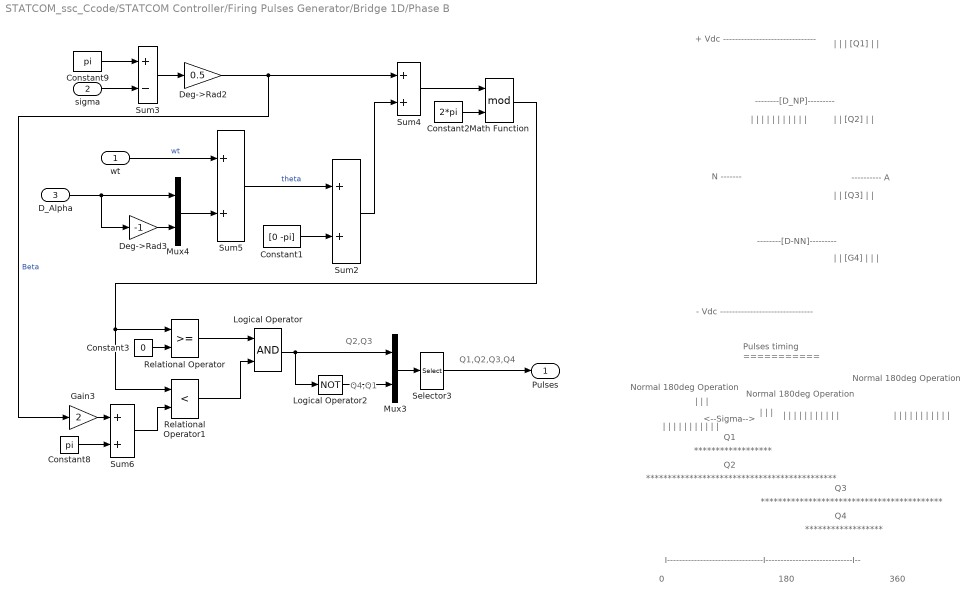
== system STATCOM_ssc_Ccode/STATCOM Controller/Firing Pulses Generator/Bridge 1D/Phase B ==
  note: <--Sigma-->
  note: |
      | |
      | |
  note: |
      | |
      | |
  note: Q4
  note: Q3
  note: Q2
  note: Q1
  note: ******************************************
  note: ********************************************
  note: ******************
  note: ******************
  note: 360
  note: 180
  note: 0
  note: I--------------------------------I-----------------------------I--
  note: Normal 180deg
      | Operation
  note: Normal 180deg
      | Operation
  note: Normal 180deg
      | Operation
  note: Pulses timing
      | ===========
  note: |
      | |
      | |
      | |
      | |
      | |
      | |
      | |
      | |
      | |
      | |
  note: |
      | |
      | |
      | |
      | |
      | |
      | |
      | |
      | |
      | |
      | |
  note: |
      | |
      | |
      | |
      | |
      | |
      | |
      | |
      | |
      | |
      | |
  note: Q1,Q2,Q3,Q4
  note: Q2,Q3
  note: Q4,Q1
  note: + Vdc -------------------------------
  note: - Vdc -------------------------------
  note: N -------
  note: |
      | |
      | |
      | |
      | |
      | |
      | |
      | |
      | |
      | |
      | |
  note: ---------- A
  note: --------[D-NN]---------
  note: --------[D_NP]---------
  note: |
      | |
      | [G4]
      | |
      | |
      | |
  note: |
      | |
      | [Q3]
      | |
      | |
  note: |
      | |
      | [Q2]
      | |
      | |
  note: |
      | |
      | |
      | [Q1]
      | |
      | |
  wt : Inport  PortDimensions=1
  sigma : Inport  Port=2  PortDimensions=1
  D_Alpha : Inport  Port=3  PortDimensions=1
  Constant1 : Constant  Value=[0 -pi]
  Constant2 : Constant  Value=2*pi
  Constant3 : Constant  Value=0
  Constant8 : Constant  Value=pi
  Constant9 : Constant  Value=pi
  Deg->Rad2 : Gain  Gain=0.5  SaturateOnIntegerOverflow=on  OutDataTypeStr=Inherit: Same as input  ParamDataTypeStr=Inherit: Same as input
  Deg->Rad3 : Gain  Gain=-1  SaturateOnIntegerOverflow=on  OutDataTypeStr=Inherit: Same as input  ParamDataTypeStr=Inherit: Same as input
  Gain3 : Gain  Gain=2  SaturateOnIntegerOverflow=on  OutDataTypeStr=Inherit: Same as input  ParamDataTypeStr=Inherit: Same as input
  Logical Operator : Logic
  Logical Operator2 : Logic  Operator=NOT
  Math Function : Math  Operator=mod  SignedPower=on
  Mux3 : Mux  Inputs=[2 2]
  Mux4 : Mux  Inputs=2
  Relational Operator : RelationalOperator
  Relational Operator1 : RelationalOperator  Operator=<
  Selector3 : Selector  InputPortWidth=4  IndexOptions=Index vector (dialog)  Indices=[4 1 2 3]  OutputSizes=1
  Sum{2,4..6} (4 alike) : Sum  InputSameDT=on  SaturateOnIntegerOverflow=on  OutDataTypeStr=Inherit: Same as first input
  Sum3 : Sum  Inputs=+-  InputSameDT=on  SaturateOnIntegerOverflow=on  OutDataTypeStr=Inherit: Same as first input
  Pulses : Outport  VectorParamsAs1DForOutWhenUnconnected=off
  wires:
  Constant2/1 -> Math Function/2
  Sum5/1 -> Sum2/1  "theta"
  wt/1 -> Sum5/1  "wt"
  D_Alpha/1 -> Mux4/1, Deg->Rad3/1
  Deg->Rad3/1 -> Mux4/2
  Mux4/1 -> Sum5/2
  Math Function/1 -> Relational Operator/1, Relational Operator1/1
  Gain3/1 -> Sum6/1
  Selector3/1 -> Pulses/1
  Mux3/1 -> Selector3/1
  Logical Operator2/1 -> Mux3/2
  Logical Operator/1 -> Mux3/1, Logical Operator2/1
  Sum4/1 -> Math Function/1
  Sum2/1 -> Sum4/2
  Sum6/1 -> Relational Operator1/2
  Constant8/1 -> Sum6/2
  Deg->Rad2/1 -> Gain3/1, Sum4/1  "Beta"
  Sum3/1 -> Deg->Rad2/1
  sigma/1 -> Sum3/2
  Constant9/1 -> Sum3/1
  Relational Operator1/1 -> Logical Operator/2
  Relational Operator/1 -> Logical Operator/1
  Constant3/1 -> Relational Operator/2
  Constant1/1 -> Sum2/2
